simulink model "Car_1_Jan_downsizewithbetteroutput"  (Simulink 8.1)
settings: Solver=ode5  StartTime=0.0  StopTime=inf  FixedStep=sample_time  RelTol=1e-3
InitFcn:
  | sample_time=0.005;%0.004;%0.0025;%0.02;
  | sample_time_Vicon = 0.005;
  | DeltaT = 0.02;
  | g = 9.81;
  | H0 = g%0.3165;
  | Kl = 1;
  | 
  | Q6_mass = 0.84;
  | 
  | Q6_Omega_r = 1.5; %for horizon ref
  | Q6_Zeta_r = 0.5; %for horizon ref
  | Q6_Omega_r_h = 2;%for vertical ref
  | Q6_Zeta_r_h = 2; %for vertical ref
  | 
  | 
  | Q6_Omega = 1.5; %for horizon control
  | Q6_Zeta = 0.5; %for horizon control
  | Q6_Omega_h= 2; %for vertical control
  | Q6_Zeta_h = 0.7; %for vertical control
  | 
  | 
  | Q6_acc_max = 5;%horizontal max acc
  | Q6_acc_max_h = 3;%horizontal max acc
  | 
  | omega_circle = 72*pi/180;
  | omega_h = 0.1;%Ascending speed
  | PI = pi;
  | Circle_R = 2.5;
  | MAX_Height = -2;
undefined symbols (not defined in the file or in its folder): DiscIntNeverNeededParam, fdesignblkfcn, gcbh
libraries: simulink x12, X330_Control x3
(part 1 of 2)
settings Model: Creator=ttcl3  LastModifiedBy=eric
settings SolverCC: MaxConsecutiveMinStep=auto
settings DebuggingCC: MultiTaskRateTransMsg=warning  FcnCallInpInsideContextMsg=EnableAllAsWarning
settings SFSimCC: SimParseCustomCode=off

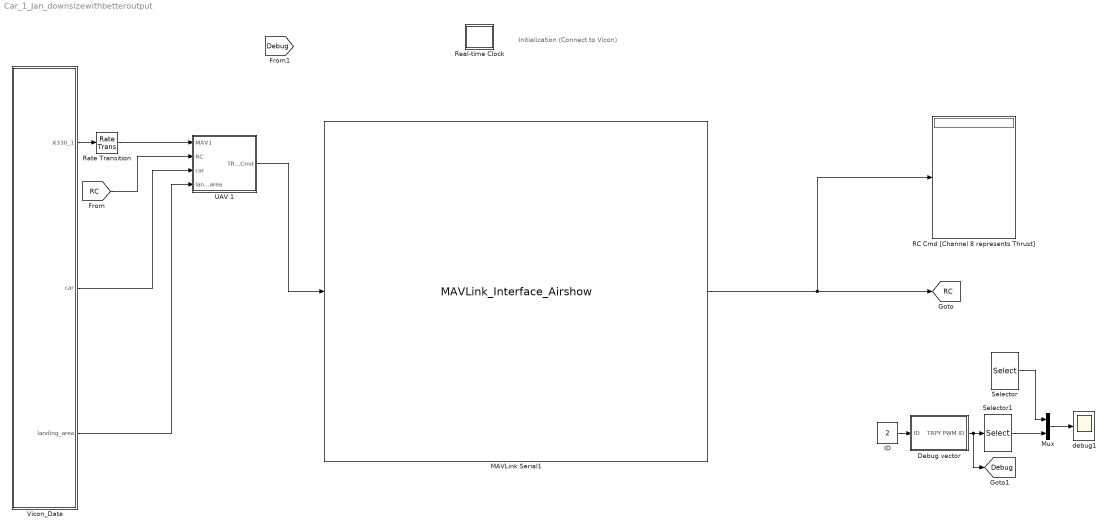
== system Car_1_Jan_downsizewithbetteroutput ==
  note: Initialization
      | (Connect to Vicon)
  Debug vector : Subsystem
  ID : Constant  Value=2
  MAVLink Serial1 : S-Function  FunctionName=MAVLink_Interface_Airshow  Parameters=COM_Port,Baud_Rate,MSG_INPUT,MSG_OUTPUT  EnableBusSupport=off  mask{COM_Port='COM5', Baud_Rate=57600, ATTITUDE_OUT=off, RC_SCALED=on, Quads_1=on, Quads_2=off, Quads_3=off, Quads_4=off, Quads_5=off, Quads_6=off}
      mask prompts: COM_Port "COM Port"; Baud_Rate "Baud Rate"; ATTITUDE_OUT "DEBUG"; RC_SCALED "RC CHANNELS SCALED"; Quads_1 "1 Quad"; Quads_2 "2 Quad"; Quads_3 "3 Quad"; Quads_4 "4 Quad"; Quads_5 "5 Quad"; Quads_6 "6 Quad"
      mask init:
      | MSG_ID_NUM_INPUT = [ uint8(221) uint8(222) uint8(223) uint8(224) uint8(225) uint8(226)];
      | MSG_ID_NAME_INPUT = [Quads_1 Quads_2 Quads_3 Quads_4 Quads_5 Quads_6];
      | 
      | MSG_ID_NUM_OUTPUT = [uint8(34) uint8(30)];
      | MSG_ID_NAME_OUTPUT = [RC_SCALED ATTITUDE_OUT ];
      | 
      | idx_input = find(MSG_ID_NAME_INPUT);
      | MSG_INPUT = MSG_ID_NUM_INPUT(idx_input);
      | 
      | idx_output = find(MSG_ID_NAME_OUTPUT);
      | MSG_OUTPUT = MSG_ID_NUM_OUTPUT(idx_output);
      mask Display:
      | % Block image
      | image(imread('10-inch Quad Heat Map.png'));
      | 
      | %Label block
      | fprintf('MAVLink Serial\n%s\n%dbps', COM_Port,  Baud_Rate)
      | 
      | 
      | %Label input ports
      | 
      | in = 1;
      | if (Quads_1 == 1)
      |     port_label('input', in, 'Quads_1');
      |     in = in + 1;
      | end
      | 
      | if (Quads_2 == 1)
      |     port_label('input', in, 'Quads_2');
      |     in = in + 1;
      | end
      | 
      | if (Quads_3 == 1)
      |     port_label('input', in, 'Quads_3');
      |     in = in + 1;
      | end
      | 
      | if (Quads_4 == 1)
      |     port_label('input', in, 'Quads_4');
      |     in = in + 1;
      | end
      | 
      | if (Quads_5 == 1)
      |     port_label('input', in, 'Quads_5');
      |     in = in + 1;
      | end
      | 
      | 
      | if (Quads_6 == 1)
      |     port_label('input', in, 'Quads_6');
      |     in = in + 1;
      | end
      | %Label output ports
      | 
      | out = 1;
      | if (RC_SCALED == 1)
      |     port_label('output', out, 'RC CMD');
      |     out = out + 1;
      | end
      | 
      | if (ATTITUDE_OUT == 1)
      |     port_label('output', out, 'DEBUG');
      |     out = out + 1;
      | end
  Mux : Mux  Inputs=2
  RC Cmd [Channel 8 represents Thrust] : Display
  Rate Transition : RateTransition  OutPortSampleTime=0.02
  Real-time Clock : Subsystem  mask(Real-time Clock){sample_time=0.02, tolerance=1}
      mask prompts: sample_time "Synchronize with real-time every n seconds:"; tolerance "Real-time warning tolerance (seconds):"
      mask help: Real-time Synchronization Block
      mask Help: This block synchronizes simulation time with the PC real-time clock or UNIX system clock. The first dialog entry is the period at which the clock is checked to insure real-time synchronization. The second dialog entry is the number of seconds that the simulation time must be within real-time before a warning is printed.
      mask Display: plot(0,0,100,100,[40,60,60,54,54,64,69,76,82,77,81,83,83,81,78,74,70,64,57,49,41,35,32,30,30,31,34,40,47,47,40,40],[90,90,85,85,80,79,76,87,80,70,64,57,49,41,33,28,24,22,21,23,25,31,37,46,56,65,73,78,80,85,85,90],[69,53,53],[64,50,73])
  Selector : Selector  InputPortWidth=6  IndexOptions=Index vector (dialog)  Indices=[3]  OutputSizes=1
  Selector1 : Selector  InputPortWidth=6  IndexOptions=Index vector (dialog)  Indices=1  OutputSizes=1
  UAV 1 : Subsystem
  Vicon_Data : Subsystem
  debug1 : Scope
      settings: TimeRange=10  YMin=-1  YMax=1
  tag scope: Debug=global, RC=global
  wires:
  [RC] -> UAV 1/2(RC)
  Vicon_Data/1(X330_1) -> Rate Transition/1
  Rate Transition/1 -> UAV 1/1(MAV1)
  Mux/1 -> debug1/1
  Debug vector/1(TRPY PWM ID) -> Selector1/1, [Debug]
  ID/1 -> Debug vector/1(ID)
  Selector/1 -> Mux/1
  Selector1/1 -> Mux/2
  UAV 1/1(TRPY Cmd) -> MAVLink Serial1/1
  Vicon_Data/2(car) -> UAV 1/3(car)
  Vicon_Data/3(landing_area) -> UAV 1/4(landing_area)
  MAVLink Serial1/1 -> [RC], RC Cmd [Channel 8 represents Thrust]/1

== system Car_1_Jan_downsizewithbetteroutput/Debug vector ==
  note: 6x1 vector (usec, XYZRPY)
  ID : Inport
  Mux1 : Mux  Inputs=6
  PWM : Constant  Value=0
  Pitch : Constant  Value=0
  Roll : Constant  Value=0
  Sine Wave : Sin  SampleTime=0
  Thrust : Constant  Value=0
  Yaw : Constant  Value=0
  TRPY PWM ID : Outport
  wires:
  Mux1/1 -> TRPY PWM ID/1
  Roll/1 -> Mux1/2
  Pitch/1 -> Mux1/3
  Yaw/1 -> Mux1/4
  PWM/1 -> Mux1/5
  ID/1 -> Mux1/6
  Sine Wave/1 -> Mux1/1

== system Car_1_Jan_downsizewithbetteroutput/Real-time Clock ==
  Real-time Clock : S-Function  FunctionName=rtclock  Parameters=sample_time, tolerance  EnableBusSupport=off

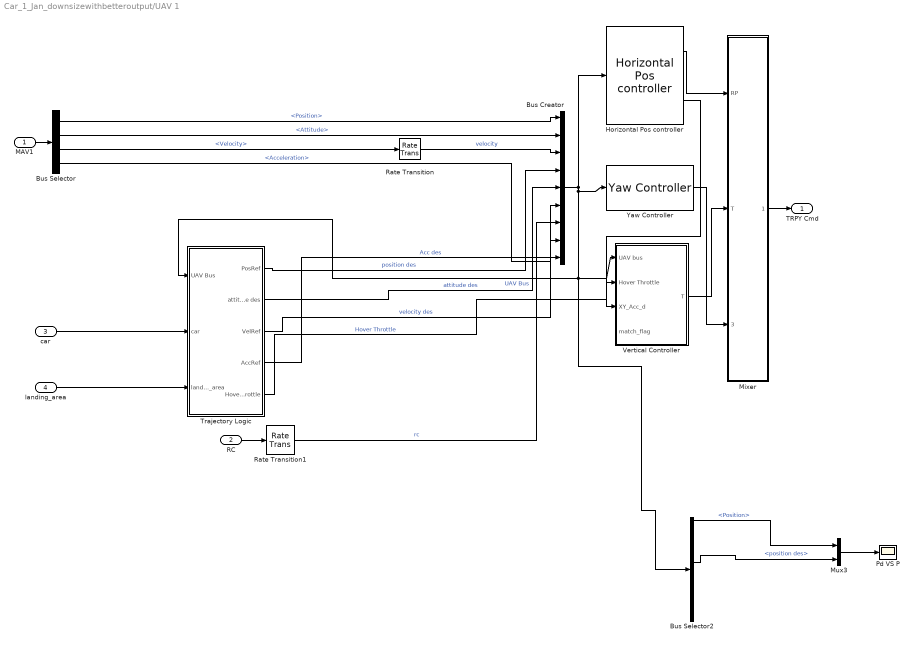
== system Car_1_Jan_downsizewithbetteroutput/UAV 1 ==
  MAV1 : Inport
  RC : Inport  Port=2
  car : Inport  Port=3
  landing_area : Inport  Port=4
  Bus Creator : BusCreator  Inputs=9
  Bus Selector : BusSelector  OutputSignals=Position,Attitude,Velocity,Acceleration
  Bus Selector2 : BusSelector  OutputSignals=Position,Attitude,velocity,position des,attitude des,velocity des,rc,Acc des
  Horizontal Pos controller : X330_Control/Horizontal Pos controller  Max_RP=60  Omega=Q6_Omega  PID_i=1  Zeta=Q6_Zeta
  Mixer : Subsystem
  Mux3 : Mux  Inputs=2
  Pd VS P : Scope
      settings: TimeRange=10  YMin=-2  YMax=1
  Rate Transition : RateTransition  OutPortSampleTime=0.02
  Rate Transition1 : RateTransition  OutPortSampleTime=0.02
  Trajectory Logic : Subsystem
  Vertical Controller : Subsystem  AncestorBlock=X330_Control/Vertical Controller  mask{Omega_h=Q6_Omega_h, Zeta_h=Q6_Zeta_h, PID_I_h=1, mass=Q6_mass}
      mask prompts: Omega_h "Omega (P Gain  = Omega^2)"; Zeta_h "Zeta (D Gain = 2*Omega*Zeta)"; PID_I_h "I Gain"
  Yaw Controller : X330_Control/Yaw Controller
  TRPY Cmd : Outport
  wires:
  Mux3/1 -> Pd VS P/1
  Bus Selector2/4 -> Mux3/2  "<position des>"
  Bus Selector2/1 -> Mux3/1  "<Position>"
  Horizontal Pos controller/2 -> Vertical Controller/3(XY_Acc_d)
  RC/1 -> Rate Transition1/1
  Trajectory Logic/4(AccRef) -> Bus Creator/9  "Acc des"
  Mixer/1(XYZ RPY) -> TRPY Cmd/1
  MAV1/1 -> Bus Selector/1
  Bus Selector/3 -> Rate Transition/1  "<Velocity>"
  Bus Selector/2 -> Bus Creator/2  "<Attitude>"
  Bus Selector/1 -> Bus Creator/1  "<Position>"
  Trajectory Logic/5(HoverThrottle) -> Vertical Controller/2(Hover Throttle)  "Hover Throttle"
  Trajectory Logic/3(VelRef) -> Bus Creator/6  "velocity des"
  Trajectory Logic/2(attitude des) -> Bus Creator/5  "attitude des"
  Trajectory Logic/1(PosRef) -> Bus Creator/4  "position des"
  Bus Selector/4 -> Bus Creator/8  "<Acceleration>"
  Vertical Controller/1(T) -> Mixer/2(T)
  Yaw Controller/1 -> Mixer/3(Yaw rate)
  Bus Creator/1 -> Yaw Controller/1, Bus Selector2/1, Vertical Controller/1(UAV bus), Trajectory Logic/1(UAV Bus), Horizontal Pos controller/1  "UAV Bus"
  Rate Transition1/1 -> Bus Creator/7  "rc"
  Rate Transition/1 -> Bus Creator/3  "velocity"
  Horizontal Pos controller/1 -> Mixer/1(RP)
  car/1 -> Trajectory Logic/2(car)
  landing_area/1 -> Trajectory Logic/3(landing_area)

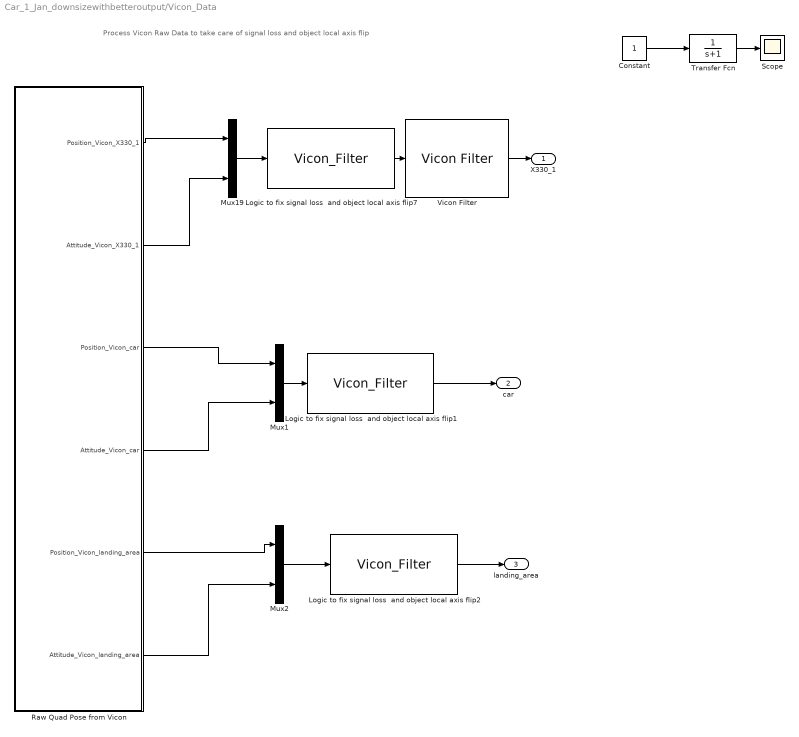
== system Car_1_Jan_downsizewithbetteroutput/Vicon_Data ==
  note: Process Vicon Raw Data to take care of signal loss and object local axis flip
  Constant : Constant  SampleTime=5
  Logic to fix signal loss  and object local axis flip1 : M-S-Function  FunctionName=Vicon_Filter
  Logic to fix signal loss  and object local axis flip2 : M-S-Function  FunctionName=Vicon_Filter
  Logic to fix signal loss  and object local axis flip7 : M-S-Function  FunctionName=Vicon_Filter
  Mux1 : Mux  Inputs=2
  Mux19 : Mux  Inputs=2
  Mux2 : Mux  Inputs=2
  Raw Quad Pose from Vicon : Subsystem
  Scope : Scope
      settings: SaveName=ScopeData2
  Transfer Fcn : TransferFcn  Denominator=[1 1]
  Vicon Filter : X330_Control/Vicon Filter
  X330_1 : Outport
  car : Outport  Port=2
  landing_area : Outport  Port=3
  wires:
  Mux19/1 -> Logic to fix signal loss  and object local axis flip7/1
  Raw Quad Pose from Vicon/1(Position_Vicon_X330_1) -> Mux19/1
  Raw Quad Pose from Vicon/2(Attitude_Vicon_X330_1) -> Mux19/2
  Logic to fix signal loss  and object local axis flip7/1 -> Vicon Filter/1
  Constant/1 -> Transfer Fcn/1
  Transfer Fcn/1 -> Scope/1
  Mux1/1 -> Logic to fix signal loss  and object local axis flip1/1
  Logic to fix signal loss  and object local axis flip1/1 -> car/1
  Raw Quad Pose from Vicon/3(Position_Vicon_car) -> Mux1/1
  Raw Quad Pose from Vicon/4(Attitude_Vicon_car) -> Mux1/2
  Mux2/1 -> Logic to fix signal loss  and object local axis flip2/1
  Logic to fix signal loss  and object local axis flip2/1 -> landing_area/1
  Raw Quad Pose from Vicon/5(Position_Vicon_landing_area) -> Mux2/1
  Raw Quad Pose from Vicon/6(Attitude_Vicon_landing_area) -> Mux2/2
  Vicon Filter/1 -> X330_1/1

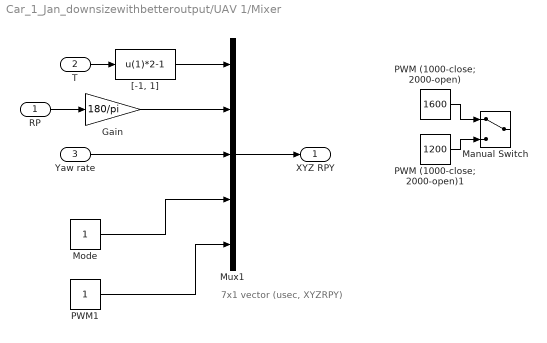
== system Car_1_Jan_downsizewithbetteroutput/UAV 1/Mixer ==
  note: 7x1 vector (usec, XYZRPY)
  RP : Inport
  T : Inport  Port=2
  Yaw rate : Inport  Port=3
  Gain : Gain  Gain=180/pi
  Manual Switch : ManualSwitch
  Mode : Constant  SampleTime=0.02
  Mux1 : Mux  Inputs=5
  PWM (1000-close; 2000-open) : Constant  Value=1600  SampleTime=0.02
  PWM (1000-close; 2000-open)1 : Constant  Value=1200  SampleTime=0.02
  PWM1 : Constant  SampleTime=0.02
  "[-1, 1]" : Fcn  Expr=u(1)*2-1
  XYZ RPY : Outport
  wires:
  "[-1, 1]"/1 -> Mux1/1
  Gain/1 -> Mux1/2
  PWM (1000-close; 2000-open)1/1 -> Manual Switch/2
  PWM (1000-close; 2000-open)/1 -> Manual Switch/1
  Yaw rate/1 -> Mux1/3
  RP/1 -> Gain/1
  T/1 -> "[-1, 1]"/1
  Mux1/1 -> XYZ RPY/1
  Mode/1 -> Mux1/4
  PWM1/1 -> Mux1/5

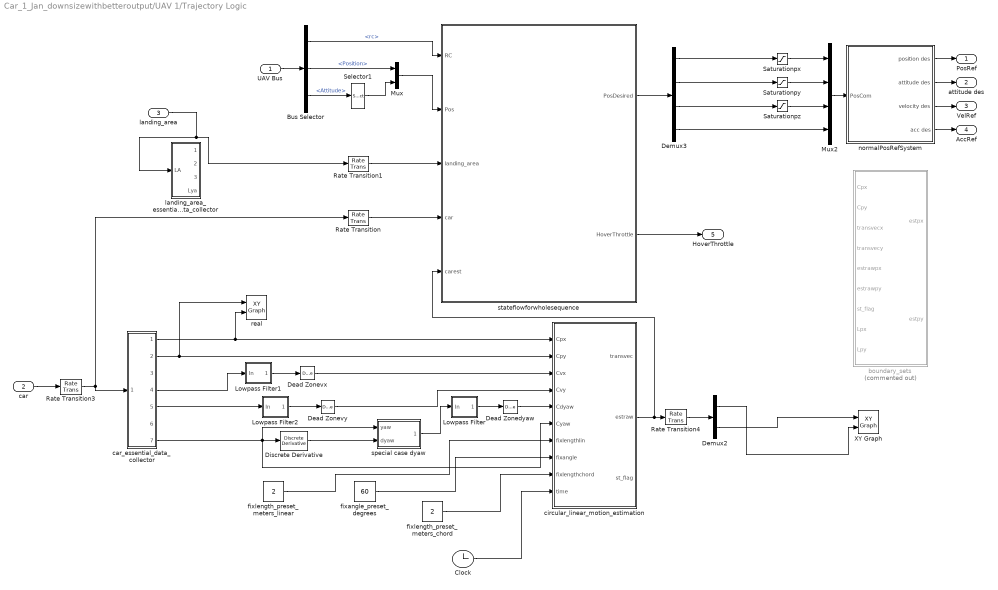
== system Car_1_Jan_downsizewithbetteroutput/UAV 1/Trajectory Logic ==
  UAV Bus : Inport
  car : Inport  Port=2
  landing_area : Inport  Port=3
  Bus Selector : BusSelector  OutputSignals=rc,Position,Attitude
  Clock : Clock
  Dead Zonedyaw : DeadZone  LowerValue=-0.6  UpperValue=0.6  SaturateOnIntegerOverflow=on
  Dead Zonevx : DeadZone  LowerValue=-0.1  UpperValue=0.1  SaturateOnIntegerOverflow=on
  Dead Zonevy : DeadZone  LowerValue=-0.1  UpperValue=0.1  SaturateOnIntegerOverflow=on
  Demux2 : Demux  Outputs=2
  Demux3 : Demux
  Discrete Derivative : simulink/Discrete/Discrete Derivative  gainval=1.0  ICPrevScaledInput=0.0  InputProcessing=Inherited  OutMin=[]  OutMax=[]  OutDataType=fixdt(1, 16)  OutScaling=2^-10  DoSatur=off
  Lowpass Filter : Subsystem  DialogController=fdesignblkfcn  DialogControllerArgs=DataTag1  InitFcn=fdesignblkfcn(gcbh, {'InitFcn'});  mask(Lowpass Filter){}
      mask help: Design a lowpass filter
      settings: CopyFcn=fdesignblkfcn(gcbh, {'CopyFcn'});
      mask Help: helpview(mapfilelocation('dsp'), 'dsplowpassfilter');
      mask Display: disp('Lowpass')
  Lowpass Filter1 : Subsystem  DialogController=fdesignblkfcn  DialogControllerArgs=DataTag3  InitFcn=fdesignblkfcn(gcbh, {'InitFcn'});  mask(Lowpass Filter){}
      mask help: Design a lowpass filter
      settings: CopyFcn=fdesignblkfcn(gcbh, {'CopyFcn'});
      mask Help: helpview(mapfilelocation('dsp'), 'dsplowpassfilter');
      mask Display: disp('Lowpass')
  Lowpass Filter2 : Subsystem  DialogController=fdesignblkfcn  DialogControllerArgs=DataTag5  InitFcn=fdesignblkfcn(gcbh, {'InitFcn'});  mask(Lowpass Filter){}
      mask help: Design a lowpass filter
      settings: CopyFcn=fdesignblkfcn(gcbh, {'CopyFcn'});
      mask Help: helpview(mapfilelocation('dsp'), 'dsplowpassfilter');
      mask Display: disp('Lowpass')
  Mux : Mux  Inputs=2
  Mux2 : Mux
  Rate Transition : RateTransition  OutPortSampleTime=0.02
  Rate Transition1 : RateTransition  OutPortSampleTime=0.02
  Rate Transition3 : RateTransition  OutPortSampleTime=0.005
  Rate Transition4 : RateTransition  OutPortSampleTime=0.1
  Saturationpx : Saturate  UpperLimit=3  LowerLimit=-3
  Saturationpy : Saturate  UpperLimit=3  LowerLimit=-3
  Saturationpz : Saturate  UpperLimit=0  LowerLimit=-2
  Selector1 : Selector  InputPortWidth=3  IndexOptions=Index vector (dialog)  Indices=[3]  OutputSizes=1
  XY Graph : simulink/Sinks/XY Graph  xmin=-4  xmax=4  ymin=-4  ymax=4  st=-1
  boundary_sets : MATLAB Function  Commented=on  TreatAsAtomicUnit=on
  car_essential_data_collector : Subsystem
  circular_linear_motion_estimation : MATLAB Function  TreatAsAtomicUnit=on
  fixangle_preset_degrees : Constant  Value=60
  fixlength_preset_meters_chord : Constant  Value=2
  fixlength_preset_meters_linear : Constant  Value=2
  landing_area_essential_data_collector : Subsystem
  normalPosRefSystem : Subsystem  AncestorBlock=X330_Control/PosRefSystem  mask{Omega_r=Q6_Omega_r, Zeta_r=Q6_Zeta_r, Acc_Max=Q6_acc_max, Omega_h_r=Q6_Omega_r_h, Zeta_h_r=Q6_Zeta_r_h, Acc_h_Max=Q6_acc_max_h}
      mask prompts: Omega_r "Omega_r (P Gain= Omega_r^2)"; Zeta_r "Zeta_r (D = 2*Omega_r*Zeta_r)"
  real : simulink/Sinks/XY Graph  xmin=-4  xmax=4  ymin=-4  ymax=4  st=-1
  special case dyaw : MATLAB Function  TreatAsAtomicUnit=on
  stateflowforwholesequence : Stateflow chart  TreatAsAtomicUnit=on
  PosRef : Outport
  attitude des : Outport  Port=2
  VelRef : Outport  Port=3
  AccRef : Outport  Port=4
  HoverThrottle : Outport  Port=5
  wires:
  Mux/1 -> stateflowforwholesequence/2(Pos)
  Selector1/1 -> Mux/2
  Bus Selector/3 -> Selector1/1  "<Attitude>"
  Bus Selector/2 -> Mux/1  "<Position>"
  UAV Bus/1 -> Bus Selector/1
  stateflowforwholesequence/2(HoverThrottle) -> HoverThrottle/1
  Bus Selector/1 -> stateflowforwholesequence/1(RC)  "<rc>"
  normalPosRefSystem/3(velocity des) -> VelRef/1
  normalPosRefSystem/1(position des) -> PosRef/1
  normalPosRefSystem/4(acc des) -> AccRef/1
  normalPosRefSystem/2(attitude des) -> attitude des/1
  stateflowforwholesequence/1(PosDesired) -> Demux3/1
  Demux3/1 -> Saturationpx/1
  Demux3/2 -> Saturationpy/1
  Demux3/3 -> Saturationpz/1
  Demux3/4 -> Mux2/4
  Saturationpx/1 -> Mux2/1
  Saturationpy/1 -> Mux2/2
  Saturationpz/1 -> Mux2/3
  Mux2/1 -> normalPosRefSystem/1(PosCom)
  fixangle_preset_degrees/1 -> circular_linear_motion_estimation/8(fixangle)
  car_essential_data_collector/7(Cya) -> Discrete Derivative/1, circular_linear_motion_estimation/6(Cyaw), special case dyaw/1(yaw)
  fixlength_preset_meters_linear/1 -> circular_linear_motion_estimation/7(fixlengthlin)
  landing_area/1 -> landing_area_essential_data_collector/1(LA), Rate Transition1/1
  car_essential_data_collector/4(CVX) -> Lowpass Filter1/1(In)
  car_essential_data_collector/5(CVY) -> Lowpass Filter2/1(In)
  Rate Transition1/1 -> stateflowforwholesequence/3(landing_area)
  Rate Transition/1 -> stateflowforwholesequence/4(car)
  car_essential_data_collector/1(CPX) -> real/2, circular_linear_motion_estimation/1(Cpx)
  car_essential_data_collector/2(CPY) -> real/1, circular_linear_motion_estimation/2(Cpy)
  Clock/1 -> circular_linear_motion_estimation/10(time)
  car/1 -> Rate Transition3/1
  Rate Transition3/1 -> Rate Transition/1, car_essential_data_collector/1(car)
  special case dyaw/1(outdyaw) -> Lowpass Filter/1(In)
  Lowpass Filter/1(Out) -> Dead Zonedyaw/1
  Lowpass Filter1/1(Out) -> Dead Zonevx/1
  Lowpass Filter2/1(Out) -> Dead Zonevy/1
  Demux2/2 -> XY Graph/1
  Demux2/1 -> XY Graph/2
  Discrete Derivative/1 -> special case dyaw/2(dyaw)
  Dead Zonedyaw/1 -> circular_linear_motion_estimation/5(Cdyaw)
  Dead Zonevx/1 -> circular_linear_motion_estimation/3(Cvx)
  Dead Zonevy/1 -> circular_linear_motion_estimation/4(Cvy)
  fixlength_preset_meters_chord/1 -> circular_linear_motion_estimation/9(fixlengthchord)
  circular_linear_motion_estimation/2(estraw) -> stateflowforwholesequence/5(carest), Rate Transition4/1
  Rate Transition4/1 -> Demux2/1

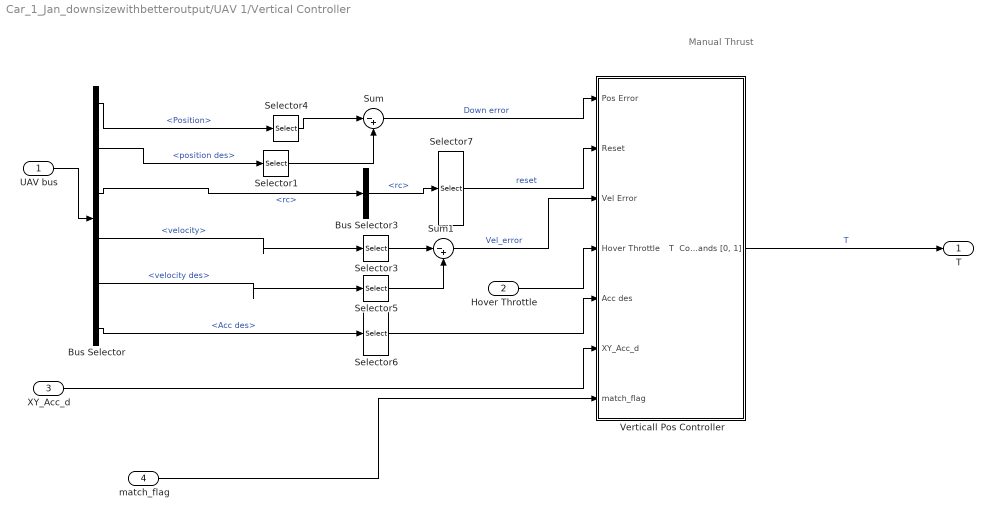
== system Car_1_Jan_downsizewithbetteroutput/UAV 1/Vertical Controller ==
  note: Manual Thrust
  UAV bus : Inport
  Hover Throttle : Inport  Port=2
  XY_Acc_d : Inport  Port=3
  match_flag : Inport  Port=4
  Bus Selector : BusSelector  OutputSignals=Position,position des,rc,velocity,velocity des,Acc des
  Bus Selector3 : BusSelector  OutputSignals=rc
  Selector{1,3..5} (4 alike) : Selector  InputPortWidth=3  IndexOptions=Index vector (dialog)  Indices=[3]  OutputSizes=1
  Selector6 : Selector  InputPortWidth=4  IndexOptions=Index vector (dialog)  Indices=[3]  OutputSizes=1
  Selector7 : Selector  InputPortWidth=8  IndexOptions=Index vector (dialog)  Indices=[7]  OutputSizes=1
  Sum : Sum  Inputs=|-+
  Sum1 : Sum  Inputs=|-+
  Verticall Pos Controller : Subsystem
  T : Outport
  wires:
  XY_Acc_d/1 -> Verticall Pos Controller/6(XY_Acc_d)
  Verticall Pos Controller/1("T  Commands [0, 1]") -> T/1  "T"
  Selector6/1 -> Verticall Pos Controller/5(Acc des)
  Bus Selector/6 -> Selector6/1  "<Acc des>"
  Hover Throttle/1 -> Verticall Pos Controller/4(Hover Throttle)
  Bus Selector/5 -> Selector5/1  "<velocity des>"
  Bus Selector/4 -> Selector3/1  "<velocity>"
  Selector5/1 -> Sum1/2
  Selector3/1 -> Sum1/1
  Sum1/1 -> Verticall Pos Controller/3(Vel Error)  "Vel_error"
  Selector7/1 -> Verticall Pos Controller/2(Reset)  "reset"
  Bus Selector3/1 -> Selector7/1  "<rc>"
  Selector1/1 -> Sum/2
  Selector4/1 -> Sum/1
  Sum/1 -> Verticall Pos Controller/1(Pos Error)  "Down error"
  Bus Selector/2 -> Selector1/1  "<position des>"
  Bus Selector/1 -> Selector4/1  "<Position>"
  Bus Selector/3 -> Bus Selector3/1  "<rc>"
  UAV bus/1 -> Bus Selector/1
  match_flag/1 -> Verticall Pos Controller/7(match_flag)

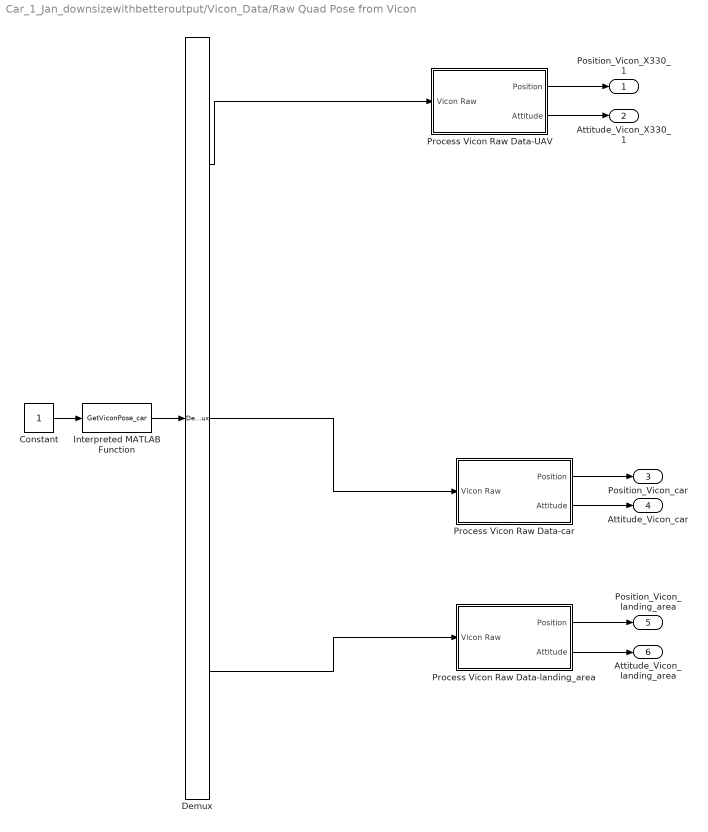
== system Car_1_Jan_downsizewithbetteroutput/Vicon_Data/Raw Quad Pose from Vicon ==
  Constant : Constant  SampleTime=sample_time
  Demux : Demux  Outputs=3
  Interpreted MATLAB Function : MATLABFcn  MATLABFcn=GetViconPose_car  OutputDimensions=18
  Process Vicon Raw Data-UAV : Subsystem
  Process Vicon Raw Data-car : Subsystem
  Process Vicon Raw Data-landing_area : Subsystem
  Position_Vicon_X330_1 : Outport
  Attitude_Vicon_X330_1 : Outport  Port=2
  Position_Vicon_car : Outport  Port=3
  Attitude_Vicon_car : Outport  Port=4
  Position_Vicon_landing_area : Outport  Port=5
  Attitude_Vicon_landing_area : Outport  Port=6
  wires:
  Interpreted MATLAB Function/1 -> Demux/1
  Process Vicon Raw Data-UAV/2(Attitude) -> Attitude_Vicon_X330_1/1
  Process Vicon Raw Data-UAV/1(Position) -> Position_Vicon_X330_1/1
  Demux/1 -> Process Vicon Raw Data-UAV/1(Vicon Raw)
  Constant/1 -> Interpreted MATLAB Function/1
  Process Vicon Raw Data-car/2(Attitude) -> Attitude_Vicon_car/1
  Process Vicon Raw Data-car/1(Position) -> Position_Vicon_car/1
  Demux/2 -> Process Vicon Raw Data-car/1(Vicon Raw)
  Process Vicon Raw Data-landing_area/2(Attitude) -> Attitude_Vicon_landing_area/1
  Process Vicon Raw Data-landing_area/1(Position) -> Position_Vicon_landing_area/1
  Demux/3 -> Process Vicon Raw Data-landing_area/1(Vicon Raw)

== system Car_1_Jan_downsizewithbetteroutput/UAV 1/Trajectory Logic/Lowpass Filter ==
  In : Inport
  Generated Filter Block : DiscreteFir  Tag=BlockMethodSubSystem  Coefficients=[-0.00036036642931867239 0.0005101271240731428 0.00044818294774894284 0.00049617715825679156 0.0006024803342551191 0.0007464774663700287 0.00092060627513123662 0.0011227676900557296 0.0013528664838050014 0.0016116819150109654 0.0019002479591395127 0.0022194593924135262 0.002570256645276354 0.0029535033116077991 0.0033695967094298667 0.0038187298509015717 0.004301098214683898 0.0048164177865245086 0.0053639103357065697 0.0059427766618668151 0.0065518958893358605 0.0071895526303495071 0.0078540155224406261 0.0085430912049437573 0.0092545967025307579 0.0099849005728561598 0.010733061231281153 0.011492647051129873 0.012262736056838865 0.013039029824582252 0.013816221907810716 0.014590906043941226 0.015359598128392602 0.016117617109568584 0.016860132245348901 0.017582743750192448 0.018281176509918829 0.018951168558931933 0.019588426713680156 0.020188702459880671 0.020748178810419252 0.021263338783452424 0.021730523601578552 0.022146416026271529 0.022508503454056819 0.022814311703779677 0.023061304941941072 0.02324808039915488 0.023373496122589675 0.023436248019836431 0.023436248019836431 0.023373496122589675 0.02324808039915488 0.023061304941941072 0.022814311703779677 0.022508503454056819 0.022146416026271529 0.021730523601578552 0.021263338783452424 0.020748178810419252 0.020188702459880671 0.019588426713680156 0.018951168558931933 0.018281176509918829 0.017582743750192448 0.016860132245348901 0.016117617109568584 0.015359598128392602 0.014590906043941226 0.013816221907810716 0.013039029824582252 0.012262736056838865 0.011492647051129873 0.010733061231281153 0.0099849005728561598 0.0092545967025307579 0.0085430912049437573 0.0078540155224406261 0.0071895526303495071 0.0065518958893358605 0.0059427766618668151 0.0053639103357065697 0.0048164177865245086 0.004301098214683898 0.0038187298509015717 0.0033695967094298667 0.0029535033116077991 0.002570256645276354 0.0022194593924135262 0.0019002479591395127 0.0016116819150109654 0.0013528664838050014 0.0011227676900557296 0.00092060627513123662 0.0007464774663700287 0.0006024803342551191 0.00049617715825679156 0.00044818294774894284 0.0005101271240731428 -0.00036036642931867239]  InputProcessing=Columns as channels (frame based)
  Out : Outport
  wires:
  In/1 -> Generated Filter Block/1
  Generated Filter Block/1 -> Out/1

== system Car_1_Jan_downsizewithbetteroutput/UAV 1/Trajectory Logic/Lowpass Filter1 ==
  In : Inport
  Generated Filter Block : DiscreteFir  Tag=BlockMethodSubSystem  Coefficients=[0.00079641397258134233 0.00095586955423693784 0.0014943702342707379 0.0021979002874955248 0.0030881215055418945 0.0041842772554791033 0.005498055721620116 0.0070397517699786203 0.0088098130080577555 0.010803120092796652 0.013005166498094144 0.015393049529249071 0.017936380656052839 0.020595894372104163 0.023325670693559314 0.026072952596765807 0.028780678477129402 0.031389279482585186 0.033838161495307786 0.036068276444773048 0.038023625616490114 0.039653938572801785 0.040916496705601636 0.041777612865850841 0.042214144439217172 0.042214144439217172 0.041777612865850841 0.040916496705601636 0.039653938572801785 0.038023625616490114 0.036068276444773048 0.033838161495307786 0.031389279482585186 0.028780678477129402 0.026072952596765807 0.023325670693559314 0.020595894372104163 0.017936380656052839 0.015393049529249071 0.013005166498094144 0.010803120092796652 0.0088098130080577555 0.0070397517699786203 0.005498055721620116 0.0041842772554791033 0.0030881215055418945 0.0021979002874955248 0.0014943702342707379 0.00095586955423693784 0.00079641397258134233]  InputProcessing=Columns as channels (frame based)
  Out : Outport
  wires:
  Generated Filter Block/1 -> Out/1
  In/1 -> Generated Filter Block/1

== system Car_1_Jan_downsizewithbetteroutput/UAV 1/Trajectory Logic/Lowpass Filter2 ==
  In : Inport
  Generated Filter Block : DiscreteFir  Tag=BlockMethodSubSystem  Coefficients=[0.00079641397258134233 0.00095586955423693784 0.0014943702342707379 0.0021979002874955248 0.0030881215055418945 0.0041842772554791033 0.005498055721620116 0.0070397517699786203 0.0088098130080577555 0.010803120092796652 0.013005166498094144 0.015393049529249071 0.017936380656052839 0.020595894372104163 0.023325670693559314 0.026072952596765807 0.028780678477129402 0.031389279482585186 0.033838161495307786 0.036068276444773048 0.038023625616490114 0.039653938572801785 0.040916496705601636 0.041777612865850841 0.042214144439217172 0.042214144439217172 0.041777612865850841 0.040916496705601636 0.039653938572801785 0.038023625616490114 0.036068276444773048 0.033838161495307786 0.031389279482585186 0.028780678477129402 0.026072952596765807 0.023325670693559314 0.020595894372104163 0.017936380656052839 0.015393049529249071 0.013005166498094144 0.010803120092796652 0.0088098130080577555 0.0070397517699786203 0.005498055721620116 0.0041842772554791033 0.0030881215055418945 0.0021979002874955248 0.0014943702342707379 0.00095586955423693784 0.00079641397258134233]  InputProcessing=Columns as channels (frame based)
  Out : Outport
  wires:
  In/1 -> Generated Filter Block/1
  Generated Filter Block/1 -> Out/1

== system Car_1_Jan_downsizewithbetteroutput/UAV 1/Trajectory Logic/car_essential_data_collector ==
  car : Inport
  Demux : Demux  Outputs=6
  Discrete Derivative : simulink/Discrete/Discrete Derivative  gainval=1.0  ICPrevScaledInput=0.0  InputProcessing=Inherited  OutMin=[]  OutMax=[]  OutDataType=fixdt(1, 16)  OutScaling=2^-10  DoSatur=off
  Discrete Derivative1 : simulink/Discrete/Discrete Derivative  gainval=1.0  ICPrevScaledInput=0.0  InputProcessing=Inherited  OutMin=[]  OutMax=[]  OutDataType=fixdt(1, 16)  OutScaling=2^-10  DoSatur=off
  Discrete Derivative2 : simulink/Discrete/Discrete Derivative  gainval=1.0  ICPrevScaledInput=0.0  InputProcessing=Inherited  OutMin=[]  OutMax=[]  OutDataType=fixdt(1, 16)  OutScaling=2^-10  DoSatur=off
  CPX : Outport
  CPY : Outport  Port=2
  CPZ : Outport  Port=3
  CVX : Outport  Port=4
  CVY : Outport  Port=5
  CVZ : Outport  Port=6
  Cya : Outport  Port=7
  wires:
  car/1 -> Demux/1
  Demux/1 -> Discrete Derivative/1, CPX/1
  Demux/2 -> Discrete Derivative1/1, CPY/1
  Demux/3 -> Discrete Derivative2/1, CPZ/1
  Demux/6 -> Cya/1
  Discrete Derivative/1 -> CVX/1
  Discrete Derivative1/1 -> CVY/1
  Discrete Derivative2/1 -> CVZ/1

== system Car_1_Jan_downsizewithbetteroutput/UAV 1/Trajectory Logic/landing_area_essential_data_collector ==
  LA : Inport
  Demux : Demux  Outputs=6
  LPX : Outport
  LPY : Outport  Port=2
  LPZ : Outport  Port=3
  Lya : Outport  Port=4
  wires:
  LA/1 -> Demux/1
  Demux/1 -> LPX/1
  Demux/2 -> LPY/1
  Demux/3 -> LPZ/1
  Demux/6 -> Lya/1

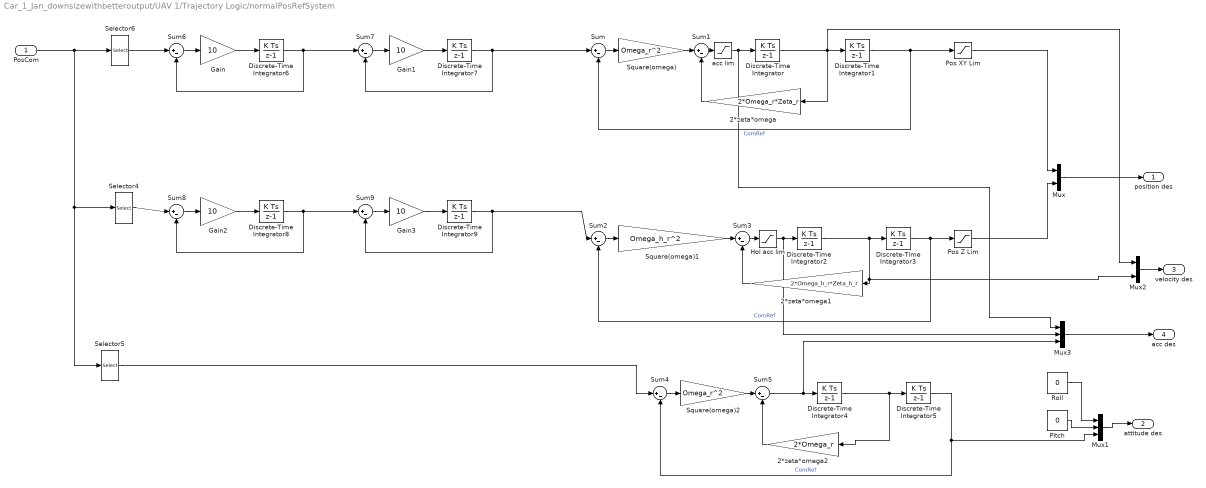
== system Car_1_Jan_downsizewithbetteroutput/UAV 1/Trajectory Logic/normalPosRefSystem ==
  PosCom : Inport
  2*zeta*omega : Gain  Gain=2*Omega_r*Zeta_r
  2*zeta*omega1 : Gain  Gain=2*Omega_h_r*Zeta_h_r
  2*zeta*omega2 : Gain  Gain=2*Omega_r
  Discrete-Time Integrator{,1..9} (10 alike) : DiscreteIntegrator  SampleTime=-1  ICPrevOutput=DiscIntNeverNeededParam  ICPrevScaledInput=DiscIntNeverNeededParam
  Gain{,1..3} (4 alike) : Gain  Gain=10
  Hol acc lim : Saturate  UpperLimit=Acc_h_Max  LowerLimit=-Acc_h_Max
  Mux : Mux  Inputs=2
  Mux1 : Mux  Inputs=3
  Mux2 : Mux  Inputs=2
  Mux3 : Mux  Inputs=3
  Pitch : Constant  Value=0  SampleTime=0.02
  Pos XY Lim : Saturate  UpperLimit=3  LowerLimit=-3
  Pos Z Lim : Saturate  LowerLimit=-1.6
  Roll : Constant  Value=0  SampleTime=0.02
  Selector4 : Selector  InputPortWidth=4  IndexOptions=Index vector (dialog)  Indices=[3]  OutputSizes=1
  Selector5 : Selector  InputPortWidth=4  IndexOptions=Index vector (dialog)  Indices=[4]  OutputSizes=1
  Selector6 : Selector  InputPortWidth=4  IndexOptions=Index vector (dialog)  Indices=[1 2]  OutputSizes=1
  Square(omega) : Gain  Gain=Omega_r^2
  Square(omega)1 : Gain  Gain=Omega_h_r^2
  Square(omega)2 : Gain  Gain=Omega_r^2
  Sum{,1..9} (10 alike) : Sum  Inputs=|+-
  acc lim : Saturate  UpperLimit=Acc_Max  LowerLimit=-Acc_Max
  position des : Outport
  attitude des : Outport  Port=2
  velocity des : Outport  Port=3
  acc des : Outport  Port=4
  wires:
  Pos Z Lim/1 -> Mux/2
  Pos XY Lim/1 -> Mux/1
  Sum9/1 -> Gain3/1
  Gain3/1 -> Discrete-Time Integrator9/1
  Discrete-Time Integrator9/1 -> Sum2/1, Sum9/2
  Sum8/1 -> Gain2/1
  Gain2/1 -> Discrete-Time Integrator8/1
  Discrete-Time Integrator8/1 -> Sum9/1, Sum8/2
  Selector4/1 -> Sum8/1
  Sum7/1 -> Gain1/1
  Gain1/1 -> Discrete-Time Integrator7/1
  Discrete-Time Integrator7/1 -> Sum/1, Sum7/2
  Sum6/1 -> Gain/1
  Gain/1 -> Discrete-Time Integrator6/1
  Discrete-Time Integrator6/1 -> Sum7/1, Sum6/2
  Selector6/1 -> Sum6/1
  Mux3/1 -> acc des/1
  Mux2/1 -> velocity des/1
  Mux1/1 -> attitude des/1
  Pitch/1 -> Mux1/2
  Roll/1 -> Mux1/1
  Mux/1 -> position des/1
  Discrete-Time Integrator1/1 -> Pos XY Lim/1, Sum/2  "ComRef"
  Selector5/1 -> Sum4/1
  2*zeta*omega2/1 -> Sum5/2
  Sum5/1 -> Mux3/3, Discrete-Time Integrator4/1
  Discrete-Time Integrator4/1 -> 2*zeta*omega2/1, Discrete-Time Integrator5/1
  Square(omega)2/1 -> Sum5/1
  Sum4/1 -> Square(omega)2/1
  Discrete-Time Integrator5/1 -> Mux1/3, Sum4/2  "ComRef"
  Hol acc lim/1 -> Mux3/2, Discrete-Time Integrator2/1
  2*zeta*omega1/1 -> Sum3/2
  Sum3/1 -> Hol acc lim/1
  Discrete-Time Integrator2/1 -> Mux2/2, 2*zeta*omega1/1, Discrete-Time Integrator3/1
  Square(omega)1/1 -> Sum3/1
  Sum2/1 -> Square(omega)1/1
  Discrete-Time Integrator3/1 -> Pos Z Lim/1, Sum2/2  "ComRef"
  acc lim/1 -> Mux3/1, Discrete-Time Integrator/1
  2*zeta*omega/1 -> Sum1/2
  Sum1/1 -> acc lim/1
  Square(omega)/1 -> Sum1/1
  Sum/1 -> Square(omega)/1
  PosCom/1 -> Selector6/1, Selector5/1, Selector4/1
  Discrete-Time Integrator/1 -> Mux2/1, 2*zeta*omega/1, Discrete-Time Integrator1/1

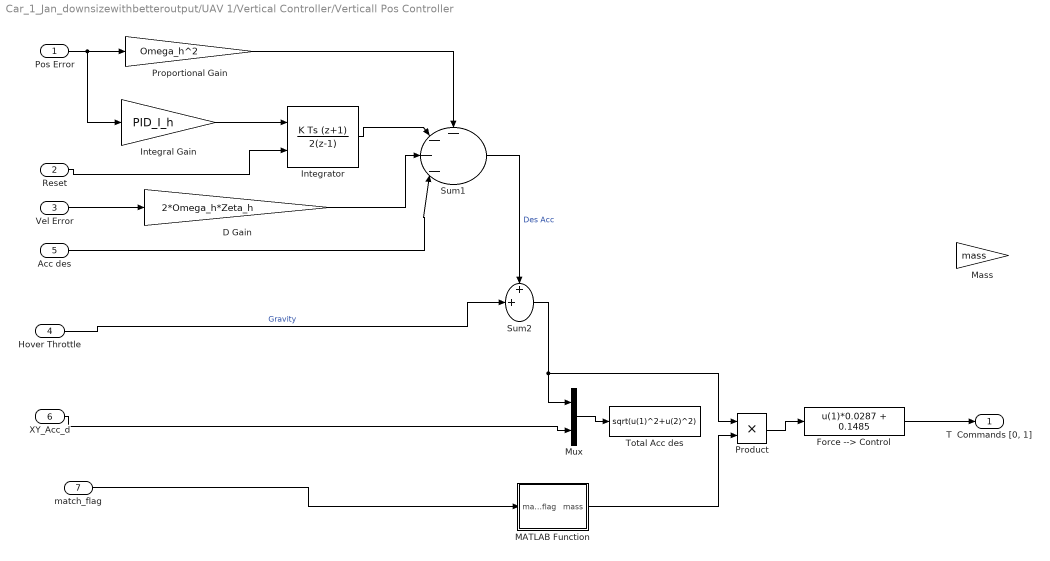
== system Car_1_Jan_downsizewithbetteroutput/UAV 1/Vertical Controller/Verticall Pos Controller ==
  Pos Error : Inport
  Reset : Inport  Port=2
  Vel Error : Inport  Port=3
  Hover Throttle : Inport  Port=4
  Acc des : Inport  Port=5
  XY_Acc_d : Inport  Port=6
  match_flag : Inport  Port=7
  D Gain : Gain  Gain=2*Omega_h*Zeta_h  OutDataTypeStr=double
  Force --> Control : Fcn  Expr=u(1)*0.0287 + 0.1485
  Integral Gain : Gain  DisableCoverage=on  Gain=PID_I_h  ParamDataTypeStr=double  OutDataTypeStr=double
  Integrator : DiscreteIntegrator  DisableCoverage=on  IntegratorMethod=Integration: Trapezoidal  ExternalReset=rising  InitialConditionMode=State only (most efficient)  SampleTime=-1  OutDataTypeStr=double  UpperSaturationLimit=0.3  LowerSaturationLimit=-0.3  ICPrevOutput=DiscIntNeverNeededParam  ICPrevScaledInput=DiscIntNeverNeededParam
  MATLAB Function : MATLAB Function  TreatAsAtomicUnit=on
  Mass : Gain  DisableCoverage=on  Gain=mass  ParamDataTypeStr=double  OutDataTypeStr=double
  Mux : Mux  Inputs=2
  Product : Product  RndMeth=Zero
  Proportional Gain : Gain  DisableCoverage=on  Gain=Omega_h^2  ParamDataTypeStr=double  OutDataTypeStr=double
  Sum1 : Sum  DisableCoverage=on  Inputs=----|  AccumDataTypeStr=double  OutDataTypeStr=double  SampleTime=0.02
  Sum2 : Sum  DisableCoverage=on  Inputs=++|  AccumDataTypeStr=double  OutDataTypeStr=double  SampleTime=0.02
  Total Acc des : Fcn  Expr=sqrt(u(1)^2+u(2)^2)
  "T  Commands [0, 1]" : Outport
  wires:
  Force --> Control/1 -> "T  Commands [0, 1]"/1
  Sum2/1 -> Product/1, Mux/1
  XY_Acc_d/1 -> Mux/2
  Mux/1 -> Total Acc des/1
  Product/1 -> Force --> Control/1
  Sum1/1 -> Sum2/1  "Des Acc"
  Hover Throttle/1 -> Sum2/2  "Gravity"
  Acc des/1 -> Sum1/4
  D Gain/1 -> Sum1/3
  Vel Error/1 -> D Gain/1
  Reset/1 -> Integrator/2
  Pos Error/1 -> Integral Gain/1, Proportional Gain/1
  Proportional Gain/1 -> Sum1/1
  Integrator/1 -> Sum1/2
  Integral Gain/1 -> Integrator/1
  match_flag/1 -> MATLAB Function/1(match_flag)
  MATLAB Function/1(mass) -> Product/2

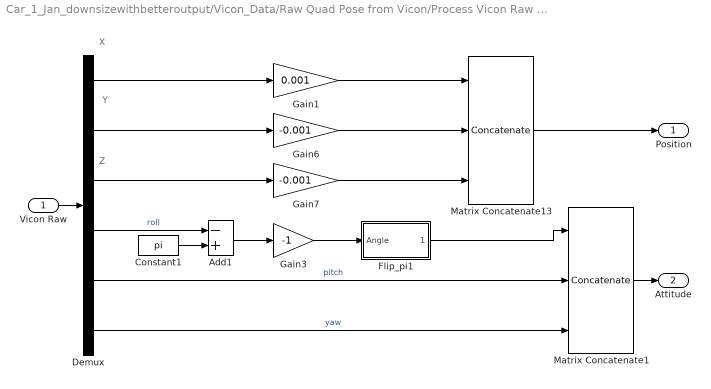
== system Car_1_Jan_downsizewithbetteroutput/Vicon_Data/Raw Quad Pose from Vicon/Process Vicon Raw Data-UAV ==
  note: X
  note: Y
  note: Z
  Vicon Raw : Inport
  Add1 : Sum  Inputs=-+
  Constant1 : Constant  Value=pi  OutDataTypeStr=double
  Demux : Demux  Outputs=6
  Flip_pi1 : Subsystem  mask(Flip -pi to pi){}
      mask help: Flips the inputs into the range -pi to pi
      mask Help: Flips the inputs into the range -pi to pi
      mask Display: disp('Flip_pi')
  Gain1 : Gain  Gain=0.001
  Gain3 : Gain  Gain=-1
  Gain6 : Gain  Gain=-0.001
  Gain7 : Gain  Gain=-0.001
  Matrix Concatenate1 : Concatenate  NumInputs=3  Mode=Multidimensional array
  Matrix Concatenate13 : Concatenate  NumInputs=3  Mode=Multidimensional array
  Position : Outport
  Attitude : Outport  Port=2
  wires:
  Constant1/1 -> Add1/2
  Demux/6 -> Matrix Concatenate1/3  "yaw"
  Gain1/1 -> Matrix Concatenate13/1
  Demux/1 -> Gain1/1
  Demux/2 -> Gain6/1
  Demux/3 -> Gain7/1
  Demux/4 -> Add1/1  "roll"
  Gain6/1 -> Matrix Concatenate13/2
  Gain7/1 -> Matrix Concatenate13/3
  Add1/1 -> Gain3/1
  Gain3/1 -> Flip_pi1/1(Angle)
  Demux/5 -> Matrix Concatenate1/2  "pitch"
  Flip_pi1/1(Angle_Flip) -> Matrix Concatenate1/1
  Matrix Concatenate13/1 -> Position/1
  Vicon Raw/1 -> Demux/1
  Matrix Concatenate1/1 -> Attitude/1

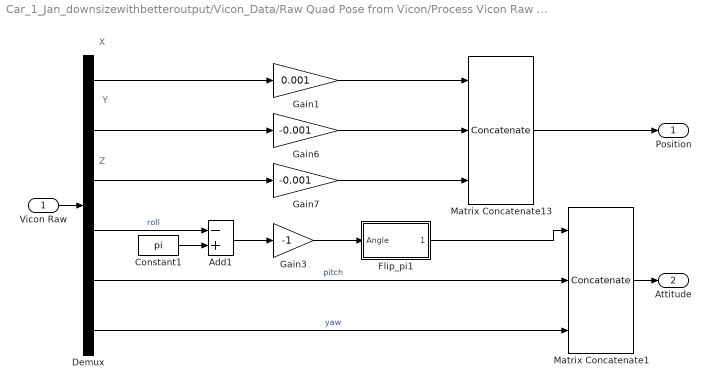
== system Car_1_Jan_downsizewithbetteroutput/Vicon_Data/Raw Quad Pose from Vicon/Process Vicon Raw Data-car ==
  note: X
  note: Y
  note: Z
  Vicon Raw : Inport
  Add1 : Sum  Inputs=-+
  Constant1 : Constant  Value=pi  OutDataTypeStr=double
  Demux : Demux  Outputs=6
  Flip_pi1 : Subsystem  mask(Flip -pi to pi){}
      mask help: Flips the inputs into the range -pi to pi
      mask Help: Flips the inputs into the range -pi to pi
      mask Display: disp('Flip_pi')
  Gain1 : Gain  Gain=0.001
  Gain3 : Gain  Gain=-1
  Gain6 : Gain  Gain=-0.001
  Gain7 : Gain  Gain=-0.001
  Matrix Concatenate1 : Concatenate  NumInputs=3  Mode=Multidimensional array
  Matrix Concatenate13 : Concatenate  NumInputs=3  Mode=Multidimensional array
  Position : Outport
  Attitude : Outport  Port=2
  wires:
  Constant1/1 -> Add1/2
  Demux/6 -> Matrix Concatenate1/3  "yaw"
  Gain1/1 -> Matrix Concatenate13/1
  Demux/1 -> Gain1/1
  Demux/2 -> Gain6/1
  Demux/3 -> Gain7/1
  Demux/4 -> Add1/1  "roll"
  Gain6/1 -> Matrix Concatenate13/2
  Gain7/1 -> Matrix Concatenate13/3
  Add1/1 -> Gain3/1
  Gain3/1 -> Flip_pi1/1(Angle)
  Demux/5 -> Matrix Concatenate1/2  "pitch"
  Flip_pi1/1(Angle_Flip) -> Matrix Concatenate1/1
  Matrix Concatenate13/1 -> Position/1
  Vicon Raw/1 -> Demux/1
  Matrix Concatenate1/1 -> Attitude/1

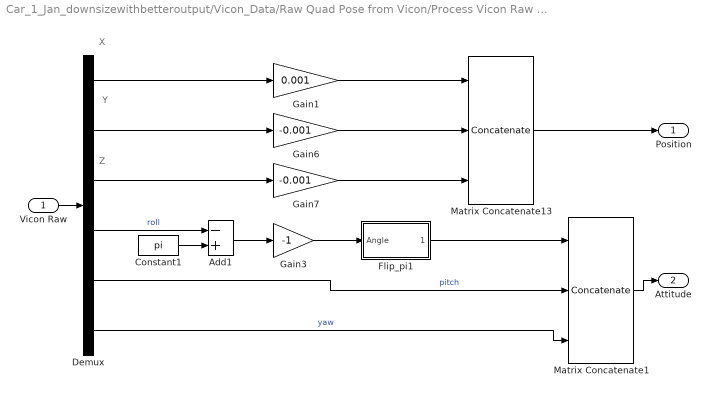
== system Car_1_Jan_downsizewithbetteroutput/Vicon_Data/Raw Quad Pose from Vicon/Process Vicon Raw Data-landing_area ==
  note: X
  note: Y
  note: Z
  Vicon Raw : Inport
  Add1 : Sum  Inputs=-+
  Constant1 : Constant  Value=pi  OutDataTypeStr=double
  Demux : Demux  Outputs=6
  Flip_pi1 : Subsystem  mask(Flip -pi to pi){}
      mask help: Flips the inputs into the range -pi to pi
      mask Help: Flips the inputs into the range -pi to pi
      mask Display: disp('Flip_pi')
  Gain1 : Gain  Gain=0.001
  Gain3 : Gain  Gain=-1
  Gain6 : Gain  Gain=-0.001
  Gain7 : Gain  Gain=-0.001
  Matrix Concatenate1 : Concatenate  NumInputs=3  Mode=Multidimensional array
  Matrix Concatenate13 : Concatenate  NumInputs=3  Mode=Multidimensional array
  Position : Outport
  Attitude : Outport  Port=2
  wires:
  Constant1/1 -> Add1/2
  Demux/6 -> Matrix Concatenate1/3  "yaw"
  Gain1/1 -> Matrix Concatenate13/1
  Demux/1 -> Gain1/1
  Demux/2 -> Gain6/1
  Demux/3 -> Gain7/1
  Demux/4 -> Add1/1  "roll"
  Gain6/1 -> Matrix Concatenate13/2
  Gain7/1 -> Matrix Concatenate13/3
  Add1/1 -> Gain3/1
  Gain3/1 -> Flip_pi1/1(Angle)
  Demux/5 -> Matrix Concatenate1/2  "pitch"
  Flip_pi1/1(Angle_Flip) -> Matrix Concatenate1/1
  Matrix Concatenate13/1 -> Position/1
  Vicon Raw/1 -> Demux/1
  Matrix Concatenate1/1 -> Attitude/1

== system Car_1_Jan_downsizewithbetteroutput/Vicon_Data/Raw Quad Pose from Vicon/Process Vicon Raw Data-UAV/Flip_pi1 ==
  Angle : Inport
  Add : Sum  Inputs=-+
  Compare To Constant1 : simulink/Logic and Bit Operations/Compare To Constant  relop=>  const=pi  OutDataTypeStr=uint8  ZeroCross=off
  Constant : Constant  Value=2*pi
  Data Type Duplicate : DataTypeDuplicate
  Flip_0_to_2pi : Subsystem  mask(Flip zero to 2pi){}
      mask help: Flips the inputs into the range zero to +2pi
      mask Help: Flips the inputs into the range zero to +2pi
      mask Display: disp('Flip_0_2pi')
  Switch : Switch  Criteria=u2 ~= 0
  Angle_Flip : Outport
  wires:
  Switch/1 -> Data Type Duplicate/1, Angle_Flip/1
  Add/1 -> Switch/1
  Constant/1 -> Add/1
  Compare To Constant1/1 -> Switch/2
  Flip_0_to_2pi/1(Angle_Flip) -> Add/2, Compare To Constant1/1, Switch/3
  Angle/1 -> Data Type Duplicate/2, Flip_0_to_2pi/1(Angle)

== system Car_1_Jan_downsizewithbetteroutput/Vicon_Data/Raw Quad Pose from Vicon/Process Vicon Raw Data-car/Flip_pi1 ==
  Angle : Inport
  Add : Sum  Inputs=-+
  Compare To Constant1 : simulink/Logic and Bit Operations/Compare To Constant  relop=>  const=pi  OutDataTypeStr=uint8  ZeroCross=off
  Constant : Constant  Value=2*pi
  Data Type Duplicate : DataTypeDuplicate
  Flip_0_to_2pi : Subsystem  mask(Flip zero to 2pi){}
      mask help: Flips the inputs into the range zero to +2pi
      mask Help: Flips the inputs into the range zero to +2pi
      mask Display: disp('Flip_0_2pi')
  Switch : Switch  Criteria=u2 ~= 0
  Angle_Flip : Outport
  wires:
  Switch/1 -> Data Type Duplicate/1, Angle_Flip/1
  Add/1 -> Switch/1
  Constant/1 -> Add/1
  Compare To Constant1/1 -> Switch/2
  Flip_0_to_2pi/1(Angle_Flip) -> Add/2, Compare To Constant1/1, Switch/3
  Angle/1 -> Data Type Duplicate/2, Flip_0_to_2pi/1(Angle)

== system Car_1_Jan_downsizewithbetteroutput/Vicon_Data/Raw Quad Pose from Vicon/Process Vicon Raw Data-landing_area/Flip_pi1 ==
  Angle : Inport
  Add : Sum  Inputs=-+
  Compare To Constant1 : simulink/Logic and Bit Operations/Compare To Constant  relop=>  const=pi  OutDataTypeStr=uint8  ZeroCross=off
  Constant : Constant  Value=2*pi
  Data Type Duplicate : DataTypeDuplicate
  Flip_0_to_2pi : Subsystem  mask(Flip zero to 2pi){}
      mask help: Flips the inputs into the range zero to +2pi
      mask Help: Flips the inputs into the range zero to +2pi
      mask Display: disp('Flip_0_2pi')
  Switch : Switch  Criteria=u2 ~= 0
  Angle_Flip : Outport
  wires:
  Switch/1 -> Data Type Duplicate/1, Angle_Flip/1
  Add/1 -> Switch/1
  Constant/1 -> Add/1
  Compare To Constant1/1 -> Switch/2
  Flip_0_to_2pi/1(Angle_Flip) -> Add/2, Compare To Constant1/1, Switch/3
  Angle/1 -> Data Type Duplicate/2, Flip_0_to_2pi/1(Angle)

== system Car_1_Jan_downsizewithbetteroutput/Vicon_Data/Raw Quad Pose from Vicon/Process Vicon Raw Data-UAV/Flip_pi1/Flip_0_to_2pi ==
  Angle : Inport
  Add : Sum
  Compare To Constant1 : simulink/Logic and Bit Operations/Compare To Constant  relop=<  const=0  OutDataTypeStr=uint8  ZeroCross=off
  Constant : Constant  Value=2*pi
  Data Type Duplicate : DataTypeDuplicate
  Flip_2pi : Subsystem  mask(Flip -2pi to 2pi){}
      mask help: Flips the inputs into the range -2pi to +2pi
      mask Help: Flips the inputs into the range -2pi to +2pi
      mask Display: disp('Flip_2pi')
  Switch : Switch  Criteria=u2 ~= 0
  Angle_Flip : Outport
  wires:
  Switch/1 -> Data Type Duplicate/1, Angle_Flip/1
  Angle/1 -> Data Type Duplicate/2, Flip_2pi/1(Angle)
  Add/1 -> Switch/1
  Constant/1 -> Add/1
  Compare To Constant1/1 -> Switch/2
  Flip_2pi/1(Angle_Flip) -> Switch/3, Add/2, Compare To Constant1/1

== system Car_1_Jan_downsizewithbetteroutput/Vicon_Data/Raw Quad Pose from Vicon/Process Vicon Raw Data-car/Flip_pi1/Flip_0_to_2pi ==
  Angle : Inport
  Add : Sum
  Compare To Constant1 : simulink/Logic and Bit Operations/Compare To Constant  relop=<  const=0  OutDataTypeStr=uint8  ZeroCross=off
  Constant : Constant  Value=2*pi
  Data Type Duplicate : DataTypeDuplicate
  Flip_2pi : Subsystem  mask(Flip -2pi to 2pi){}
      mask help: Flips the inputs into the range -2pi to +2pi
      mask Help: Flips the inputs into the range -2pi to +2pi
      mask Display: disp('Flip_2pi')
  Switch : Switch  Criteria=u2 ~= 0
  Angle_Flip : Outport
  wires:
  Switch/1 -> Data Type Duplicate/1, Angle_Flip/1
  Angle/1 -> Data Type Duplicate/2, Flip_2pi/1(Angle)
  Add/1 -> Switch/1
  Constant/1 -> Add/1
  Compare To Constant1/1 -> Switch/2
  Flip_2pi/1(Angle_Flip) -> Switch/3, Add/2, Compare To Constant1/1

== system Car_1_Jan_downsizewithbetteroutput/Vicon_Data/Raw Quad Pose from Vicon/Process Vicon Raw Data-landing_area/Flip_pi1/Flip_0_to_2pi ==
  Angle : Inport
  Add : Sum
  Compare To Constant1 : simulink/Logic and Bit Operations/Compare To Constant  relop=<  const=0  OutDataTypeStr=uint8  ZeroCross=off
  Constant : Constant  Value=2*pi
  Data Type Duplicate : DataTypeDuplicate
  Flip_2pi : Subsystem  mask(Flip -2pi to 2pi){}
      mask help: Flips the inputs into the range -2pi to +2pi
      mask Help: Flips the inputs into the range -2pi to +2pi
      mask Display: disp('Flip_2pi')
  Switch : Switch  Criteria=u2 ~= 0
  Angle_Flip : Outport
  wires:
  Switch/1 -> Data Type Duplicate/1, Angle_Flip/1
  Angle/1 -> Data Type Duplicate/2, Flip_2pi/1(Angle)
  Add/1 -> Switch/1
  Constant/1 -> Add/1
  Compare To Constant1/1 -> Switch/2
  Flip_2pi/1(Angle_Flip) -> Switch/3, Add/2, Compare To Constant1/1

== system Car_1_Jan_downsizewithbetteroutput/Vicon_Data/Raw Quad Pose from Vicon/Process Vicon Raw Data-UAV/Flip_pi1/Flip_0_to_2pi/Flip_2pi ==
  Angle : Inport
  Bias : Bias  Bias=-2*pi
  Constant : Constant  Value=2*pi
  Data Type Duplicate : DataTypeDuplicate
  Modulo : Math  Operator=mod  SaturateOnIntegerOverflow=on
  Sign1 : Signum
  Switch : Switch
  Angle_Flip : Outport
  wires:
  Switch/1 -> Data Type Duplicate/2, Angle_Flip/1
  Bias/1 -> Switch/3
  Sign1/1 -> Switch/2
  Modulo/1 -> Switch/1, Bias/1
  Constant/1 -> Modulo/2
  Angle/1 -> Data Type Duplicate/1, Sign1/1, Modulo/1

== system Car_1_Jan_downsizewithbetteroutput/Vicon_Data/Raw Quad Pose from Vicon/Process Vicon Raw Data-car/Flip_pi1/Flip_0_to_2pi/Flip_2pi ==
  Angle : Inport
  Bias : Bias  Bias=-2*pi
  Constant : Constant  Value=2*pi
  Data Type Duplicate : DataTypeDuplicate
  Modulo : Math  Operator=mod  SaturateOnIntegerOverflow=on
  Sign1 : Signum
  Switch : Switch
  Angle_Flip : Outport
  wires:
  Switch/1 -> Data Type Duplicate/2, Angle_Flip/1
  Bias/1 -> Switch/3
  Sign1/1 -> Switch/2
  Modulo/1 -> Switch/1, Bias/1
  Constant/1 -> Modulo/2
  Angle/1 -> Data Type Duplicate/1, Sign1/1, Modulo/1

== system Car_1_Jan_downsizewithbetteroutput/Vicon_Data/Raw Quad Pose from Vicon/Process Vicon Raw Data-landing_area/Flip_pi1/Flip_0_to_2pi/Flip_2pi ==
  Angle : Inport
  Bias : Bias  Bias=-2*pi
  Constant : Constant  Value=2*pi
  Data Type Duplicate : DataTypeDuplicate
  Modulo : Math  Operator=mod  SaturateOnIntegerOverflow=on
  Sign1 : Signum
  Switch : Switch
  Angle_Flip : Outport
  wires:
  Switch/1 -> Data Type Duplicate/2, Angle_Flip/1
  Bias/1 -> Switch/3
  Sign1/1 -> Switch/2
  Modulo/1 -> Switch/1, Bias/1
  Constant/1 -> Modulo/2
  Angle/1 -> Data Type Duplicate/1, Sign1/1, Modulo/1

== matlab function UAV 1/Trajectory Logic/circular_linear_motion_estimation ==
  data: Cpx input double; Cpy input double; Cvx input double; Cvy input double; Cdyaw input double; Cyaw input double; fixlengthlin input double; transvec output double; estraw output double; fixangle input double; fixlengthchord input double; st_flag output double; time input double
function [transvec,estraw,st_flag] = fcn(Cpx,Cpy,Cvx,Cvy,Cdyaw,Cyaw,fixlengthlin,fixangle,fixlengthchord,time)
if(Cvx == 0 && Cvy == 0)
    st_flag = 1;
else 
    st_flag = 0;
end
%%%%%%%%%%%%%%%%%%%%%%circular estimation%%%%%%%%%%%%%%%%%%%%%%%%%%%%
vxyM = sqrt((Cvx)^2 + (Cvy)^2); %resultant vector vxy
if(st_flag == 0)
    
        angleOmega = acos(abs(Cvx)/vxyM) + 0.5 * fixangle * pi / 180; %angleOmega(radian): between vx and L
        zero_chk = 1;
else
    
      angleOmega = 0;  
      zero_chk = 0;
end
if(Cdyaw ~= 0) %use dyaw to select circular or linear estimation
%r = vxyM / abs(Cdyaw);
%Chord = 2 * r * sin(fixangle * pi / 360); %%%%%chord sometime will go to
%very large value, will disable this parameter soon
transveccir = [fixlengthchord * cos(angleOmega)*zero_chk  fixlengthchord * sin(angleOmega) * zero_chk];
transveclin = [0 0];
else
%%%%%%%%%%%%%%%%%%%%%%%%linear estimation%%%%%%%%%%%%%%%%%%%%%%%%%%%%%%
transveclin = [fixlengthlin * cos(Cyaw * pi / 180)*zero_chk fixlengthlin * sin(Cyaw * pi / 180)*zero_chk];
transveccir = [0 0];
%Chord = 0;
end
if(time<2)       %%%%%%%%%%%%%%%%%avoid noise when initializing the program in first 2 seconds
    transvec = [0 0];
else
transvec = transveccir + transveclin;
end

C2dvec = [Cpx Cpy];
estraw = C2dvec + transvec;

== matlab function UAV 1/Trajectory Logic/boundary_sets ==
  data: Cpx input double; Cpy input double; transvecx input double; transvecy input double; estrawpx input double; estrawpy input double; st_flag input double; estpx output double; Lpx input double; Lpy input double; estpy output double
function [estpx,estpy] = fcn(Cpx,Cpy,transvecx,transvecy,estrawpx,estrawpy,st_flag,Lpx,Lpy)
%%%%%%%%%%%%%%%%%%%landing_area check and avoidance%%%%%%%%%%%%%%%%%%%%%%%%%%%
transvecM = sqrt(transvecx^2 + transvecy^2);
if(st_flag == 0)
unitransvecx = transvecx / transvecM; %%calculate unit vector for transvector
unitransvecy = transvecy / transvecM;
else
unitransvecx = 0; %%calculate unit vector for transvector
unitransvecy = 0;
end
%%%%%%%%%%%%%%%%%%%%%%%%%%%%%%%%%%%%%%%%%%%%%%%%%%%%%%%%%%%%%%%%%%%%%%%%%%%
disLx = Lpx - estrawpx;
disLy = Lpy - estrawpy;
disLM = sqrt((disLx)^2 + (disLy)^2);
if(disLM <= 1.2)
while(disLM <= 1.2) %%%%%%%%%loop if the estimation position is in 1.2 circle area%%%%%%%%%%%%%%%
    estlooppx = estrawpx - 0.01 * unitransvecx; %% every time of loop move back reverse transvector 1mm
    estlooppy = estrawpy - 0.01 * unitransvecy;
end
    estpx = estlooppx;
    estpy = estlooppy;
else
    estpx = Cpx + transvecx;
    estpy = Cpy + transvecy;
end

== matlab function UAV 1/Trajectory Logic/special case dyaw ==
  data: yaw input double; outdyaw output double; dyaw input double
function outdyaw = fcn(yaw,dyaw)
%#codegen
if(yaw > 3 || yaw<-3)
    outdyaw = 0;
else
    outdyaw = dyaw;
end
